simulink library "amg_sense_temphumid_lib"  (R2015b)
settings: Solver=ode45  StartTime=0.0  StopTime=10.0  RelTol=1e-3
libraries: simulink x24, waijung_soft_i2c_lib x2
settings Model: Creator=Krisada  LastModifiedBy=Aimagin
settings DataIOCC: SaveFormat=Array  SignalLoggingSaveFormat=ModelDataLogs
settings OptimizationCC: ExpressionDepthLimit=2147483647
settings DebuggingCC: UnderspecifiedInitializationDetection=Classic  MergeDetectMultiDrivingBlocksExec=none  SolverPrmCheckMsg=warning  FcnCallInpInsideContextMsg=UseLocalSettings  StateNameClashWarn=warning  StrictBusMsg=Warning
settings HardwareCC: ProdBitPerPointer=32  ProdLargestAtomicFloat=None  ProdIntDivRoundTo=Undefined  ProdEndianess=Unspecified  ProdWordSize=32  ProdHWDeviceType=32-bit Generic
settings GRTTargetCC: CombineOutputUpdateFcns=off  GRTInterface=on
settings ConfigComp: CovModelRefEnable=Off

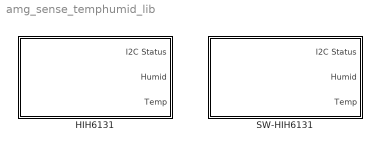
== system amg_sense_temphumid_lib ==
  HIH6131 : Subsystem  mask(stm32f4_i2c_sensors){module=1, slvaddr=hex2dec('4E'), outputlabel={'I2C Status','Humid (%)','Temp (C)'}, sensorname=STM32F4\naMG Sense - Temp/Humid, sampletime=0.5}
      mask prompts: module "I2C Module"; slvaddr "I2C Slave Address"; outputlabel "Output label"; sensorname "Sensor name"; sampletime "Sample time (sec)"
      mask help:
      | aMG Sense - Temp/Humid
      |
      | I2C Status:
      |  0 - Success
      |  1 - NAK
      |  2 - Timeout
      |  3 - Combined error, NAK+Timeout
      |
      | Note: Require I2C Setup block for the selected I2C module.
      mask init:
      | stm32f4_i2c_sensors_callback('init');
      mask TypeOptions module: 1 | 2 | 3
      mask Callback module: stm32f4_i2c_sensors_callback('module');
      mask Display: text(0.5, 0.5, 'STM32F4\naMG Sense - Temp/Humid','ver','middle','hor','center');port_label('output', 1,'I2C Status');port_label('output', 2,'Humid (%)');port_label('output', 3,'Temp (C)');
  SW-HIH6131 : Subsystem  mask(waijung_soft_i2c_sensors){module=1, slvaddr=hex2dec('4E'), outputlabel={'I2C Status','Humid (%)','Temp (C)'}, sensorname=Soft-I2C\naMG Sense - Temp/Humid, sampletime=0.5}
      mask prompts: module "I2C Module"; slvaddr "I2C Slave Address"; outputlabel "Output label"; sensorname "Sensor name"; sampletime "Sample time (sec)"
      mask help:
      | aMG Sense - Temp/Humid
      |
      | I2C Status:
      |  0 - Success
      |  1 - NAK
      |  2 - Timeout
      |  3 - Combined error, NAK+Timeout
      |
      | Note: Require I2C Setup block for the selected I2C module.
      mask init:
      | waijung_soft_i2c_sensors_callback('init');
      mask TypeOptions module: 1 | 2 | 3 | 4 | 5 | 6 | 7 | 8 | 9 | 10 | 11 | 12 | 13 | 14 | 15 | 16 | 17 | 18 | 19 | 20 | 21 | 22 | 23 | 24 | 25 | 26 | 27 | 28 | 29 | 30 | 31 | 32
      mask Callback module: waijung_soft_i2c_sensors_callback('module');
      mask Display: text(0.5, 0.5, 'Soft-I2C\naMG Sense - Temp/Humid','ver','middle','hor','center');port_label('output', 1,'I2C Status');port_label('output', 2,'Humid (%)');port_label('output', 3,'Temp (C)');

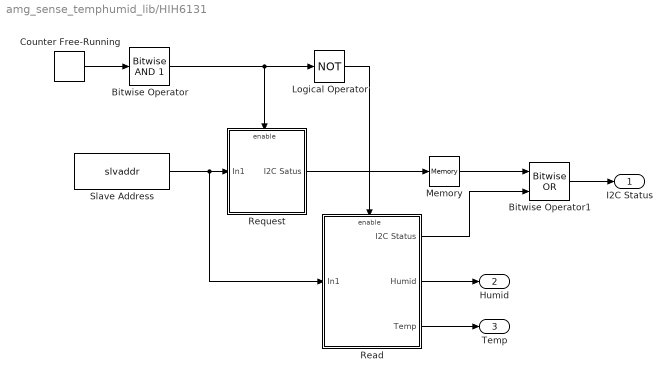
== system amg_sense_temphumid_lib/HIH6131 ==
  Bitwise Operator : simulink/Logic and Bit Operations/Bitwise Operator  logicop=AND  UseBitMask=on  BitMask=1  BitMaskRealWorld=Stored Integer
  Bitwise Operator1 : simulink/Logic and Bit Operations/Bitwise Operator  logicop=OR  UseBitMask=off  NumInputPorts=2  BitMask=bin2dec('11011001')  BitMaskRealWorld=Stored Integer
  Counter Free-Running : simulink/Sources/Counter Free-Running  SystemSampleTime=-1  NumBits=16  tsamp=-1
  Logical Operator : Logic  Operator=NOT  AllPortsSameDT=off  OutDataTypeStr=boolean
  Memory : Memory  InheritSampleTime=on  LinearizeMemory=on
  Read : Subsystem
  Request : Subsystem
  Slave Address : Constant  Value=slvaddr  OutDataTypeStr=uint8  SampleTime=sampletime
  I2C Status : Outport
  Humid : Outport  Port=2
  Temp : Outport  Port=3
  wires:
  Counter Free-Running/1 -> Bitwise Operator/1
  Bitwise Operator/1 -> Logical Operator/1, Request/Enable
  Logical Operator/1 -> Read/Enable
  Slave Address/1 -> Request/1(In1), Read/1(In1)
  Read/2(Humid) -> Humid/1
  Read/3(Temp) -> Temp/1
  Request/1(I2C Satus) -> Memory/1
  Memory/1 -> Bitwise Operator1/1
  Read/1(I2C Status) -> Bitwise Operator1/2
  Bitwise Operator1/1 -> I2C Status/1

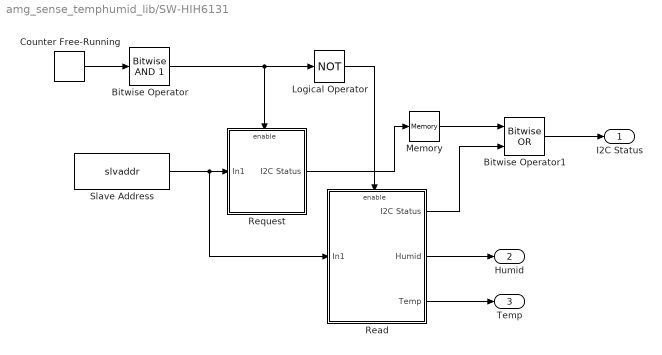
== system amg_sense_temphumid_lib/SW-HIH6131 ==
  Bitwise Operator : simulink/Logic and Bit Operations/Bitwise Operator  logicop=AND  UseBitMask=on  BitMask=1  BitMaskRealWorld=Stored Integer
  Bitwise Operator1 : simulink/Logic and Bit Operations/Bitwise Operator  logicop=OR  UseBitMask=off  NumInputPorts=2  BitMask=bin2dec('11011001')  BitMaskRealWorld=Stored Integer
  Counter Free-Running : simulink/Sources/Counter Free-Running  SystemSampleTime=-1  NumBits=16  tsamp=-1
  Logical Operator : Logic  Operator=NOT  AllPortsSameDT=off  OutDataTypeStr=boolean
  Memory : Memory  InheritSampleTime=on  LinearizeMemory=on
  Read : Subsystem
  Request : Subsystem
  Slave Address : Constant  Value=slvaddr  OutDataTypeStr=uint8  SampleTime=sampletime
  I2C Status : Outport
  Humid : Outport  Port=2
  Temp : Outport  Port=3
  wires:
  Read/3(Temp) -> Temp/1
  Read/2(Humid) -> Humid/1
  Slave Address/1 -> Read/1(In1), Request/1(In1)
  Logical Operator/1 -> Read/Enable
  Bitwise Operator/1 -> Request/Enable, Logical Operator/1
  Counter Free-Running/1 -> Bitwise Operator/1
  Request/1(I2C Status) -> Memory/1
  Memory/1 -> Bitwise Operator1/1
  Read/1(I2C Status) -> Bitwise Operator1/2
  Bitwise Operator1/1 -> I2C Status/1

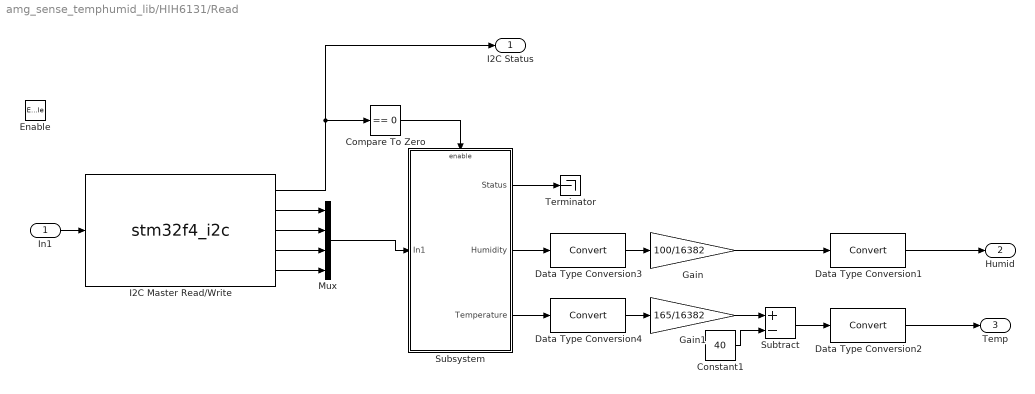
== system amg_sense_temphumid_lib/HIH6131/Read ==
  In1 : Inport
  Enable : EnablePort  PropagateVarSize=During execution
  Compare To Zero : simulink/Logic and Bit Operations/Compare To Zero  SystemSampleTime=-1  relop===  LogicOutDataTypeMode=boolean  ZeroCross=off
  Constant1 : Constant  Value=40
  Data Type Conversion{1..4} (4 alike) : DataTypeConversion
  Gain : Gain  Gain=100/16382
  Gain1 : Gain  Gain=165/16382
  I2C Master Read/Write : S-Function  FunctionName=stm32f4_i2c  Parameters=configuration,module,transfer,clkspeed,timeout,sdapin,sclpin,writecount,readcount,inputtypearray,outputtypearray,confstr,sampletime,sampletimestr,blockid  SFunctionDeploymentMode=off  EnableBusSupport=off  mask(stm32f4_i2c){configuration=Transaction, module=1, lastmodule=3, transfer=Blocking, dutycycle=TLow/THigh = 2, clkspeed=400, timeout=25, writecount=0, readcount=4, sdapin=C9, sclpin=A8, waitwritetime=0, inputtypearray=[1 3], outputtypearray=[5 3 3 3 3 3], confstr=["C","9","A","8","1","1","6","0","I2C_DutyCycle_2","0","off"], sampletime=-1, sampletimestr=0.5, blockid=ReadI2CMasterReadWrite}
      mask prompts: module "I2C Module"; lastmodule "Last module"; transfer "Transfer mode"; dutycycle "Duty cycle in fast mode"; clkspeed "Clock speed (kHz)"; timeout "Timeout (ms)"; writecount "Bytes write count"; readcount "Bytes read count"; sdapin "SDA pin"; sclpin "SCL pin"; waitwritetime "Wait write time (ms), default is 0"; inputtypearray "Input type array"; outputtypearray "Output type array"; confstr "Configuration string"; sampletime "Sample time (sec)"; sampletimestr "Compiled sample time (sec) in string"
      mask init:
      | stm32f4_i2c_callback('init');
      mask Help: web(fullfile(waijungdocroot,'stm32f4_i2c_readwrite.htm'), '-browser')
      mask TypeOptions configuration: Setup | Transaction
      mask Callback configuration: stm32f4_i2c_callback('configuration');
      mask TypeOptions module: 1 | 2 | 3
      mask Callback module: stm32f4_i2c_callback('module');
      mask TypeOptions transfer: Blocking | Non-blocking
      mask TypeOptions dutycycle: TLow/THigh = 16/9 | TLow/THigh = 2
      mask Callback dutycycle: stm32f4_i2c_callback('dutycycle');
      mask Callback writecount: stm32f4_i2c_callback('writecount');
      mask Callback readcount: stm32f4_i2c_callback('readcount');
      mask TypeOptions sdapin: - | C9
      mask Callback sdapin: stm32f4_i2c_callback('sdapin');
      mask TypeOptions sclpin: - | A8
      mask Callback sclpin: stm32f4_i2c_callback('sclpin');
      mask Callback confstr: stm32f4_i2c_callback('confstr');
      mask Callback sampletime: stm32f4_i2c_callback('sampletime');
      mask Callback sampletimestr: stm32f4_i2c_callback('sampletimestr');
      mask Callback blockid: stm32f4_i2c_callback('blockid');
      mask Display: text(0.5, 0.5, 'Module: I2C1\nTransfer: Blocking\nWrite: 0 bytes\nRead: 4 bytes\nTs (sec): 0.5','ver','middle','hor','center');port_label('input', 1,'SlvAddr');port_label('output', 1,'Status');port_label('output', 2,'Rd0 (uint8)');port_label('output', 3,'Rd1 (uint8)');port_label('output', 4,'Rd2 (uint8)');port_label('output', 5,'Rd3 (uint8)');
  Mux : Mux
  Subsystem : Subsystem
  Subtract : Sum  Inputs=+-
  Terminator : Terminator
  I2C Status : Outport
  Humid : Outport  Port=2
  Temp : Outport  Port=3
  wires:
  I2C Master Read/Write/2 -> Mux/1
  I2C Master Read/Write/3 -> Mux/2
  I2C Master Read/Write/4 -> Mux/3
  I2C Master Read/Write/5 -> Mux/4
  Mux/1 -> Subsystem/1(In1)
  Compare To Zero/1 -> Subsystem/Enable
  I2C Master Read/Write/1 -> Compare To Zero/1, I2C Status/1
  Subsystem/2(Humidity) -> Data Type Conversion3/1
  Subsystem/3(Temperature) -> Data Type Conversion4/1
  Gain1/1 -> Subtract/1
  Constant1/1 -> Subtract/2
  Subsystem/1(Status) -> Terminator/1
  Subtract/1 -> Data Type Conversion2/1
  Data Type Conversion3/1 -> Gain/1
  Data Type Conversion4/1 -> Gain1/1
  Gain/1 -> Data Type Conversion1/1
  Data Type Conversion1/1 -> Humid/1
  Data Type Conversion2/1 -> Temp/1
  In1/1 -> I2C Master Read/Write/1

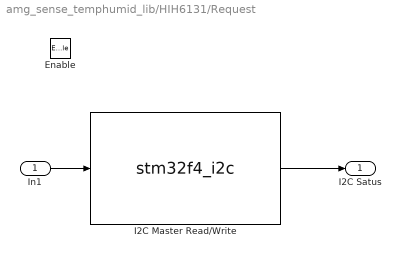
== system amg_sense_temphumid_lib/HIH6131/Request ==
  In1 : Inport
  Enable : EnablePort  PropagateVarSize=During execution
  I2C Master Read/Write : S-Function  FunctionName=stm32f4_i2c  Parameters=configuration,module,transfer,clkspeed,timeout,sdapin,sclpin,writecount,readcount,inputtypearray,outputtypearray,confstr,sampletime,sampletimestr,blockid  SFunctionDeploymentMode=off  EnableBusSupport=off  mask(stm32f4_i2c){configuration=Transaction, module=1, lastmodule=3, transfer=Blocking, dutycycle=TLow/THigh = 2, clkspeed=400, timeout=25, writecount=0, readcount=0, sdapin=C9, sclpin=A8, waitwritetime=0, inputtypearray=[1 3], outputtypearray=[1 3], confstr=["C","9","A","8","1","1","6","0","I2C_DutyCycle_2","0","off"], sampletime=-1, sampletimestr=0.5, blockid=RequestI2CMasterReadWrite}
      mask prompts: module "I2C Module"; lastmodule "Last module"; transfer "Transfer mode"; dutycycle "Duty cycle in fast mode"; clkspeed "Clock speed (kHz)"; timeout "Timeout (ms)"; writecount "Bytes write count"; readcount "Bytes read count"; sdapin "SDA pin"; sclpin "SCL pin"; waitwritetime "Wait write time (ms), default is 0"; inputtypearray "Input type array"; outputtypearray "Output type array"; confstr "Configuration string"; sampletime "Sample time (sec)"; sampletimestr "Compiled sample time (sec) in string"
      mask init:
      | stm32f4_i2c_callback('init');
      mask Help: web(fullfile(waijungdocroot,'stm32f4_i2c_readwrite.htm'), '-browser')
      mask TypeOptions configuration: Setup | Transaction
      mask Callback configuration: stm32f4_i2c_callback('configuration');
      mask TypeOptions module: 1 | 2 | 3
      mask Callback module: stm32f4_i2c_callback('module');
      mask TypeOptions transfer: Blocking | Non-blocking
      mask TypeOptions dutycycle: TLow/THigh = 16/9 | TLow/THigh = 2
      mask Callback dutycycle: stm32f4_i2c_callback('dutycycle');
      mask Callback writecount: stm32f4_i2c_callback('writecount');
      mask Callback readcount: stm32f4_i2c_callback('readcount');
      mask TypeOptions sdapin: - | C9
      mask Callback sdapin: stm32f4_i2c_callback('sdapin');
      mask TypeOptions sclpin: - | A8
      mask Callback sclpin: stm32f4_i2c_callback('sclpin');
      mask Callback confstr: stm32f4_i2c_callback('confstr');
      mask Callback sampletime: stm32f4_i2c_callback('sampletime');
      mask Callback sampletimestr: stm32f4_i2c_callback('sampletimestr');
      mask Callback blockid: stm32f4_i2c_callback('blockid');
      mask Display: text(0.5, 0.5, 'Module: I2C1\nTransfer: Blocking\nWrite: 0 bytes\nRead: 0 bytes\nTs (sec): 0.5','ver','middle','hor','center');port_label('input', 1,'SlvAddr');port_label('output', 1,'Status');
  I2C Satus : Outport
  wires:
  In1/1 -> I2C Master Read/Write/1
  I2C Master Read/Write/1 -> I2C Satus/1

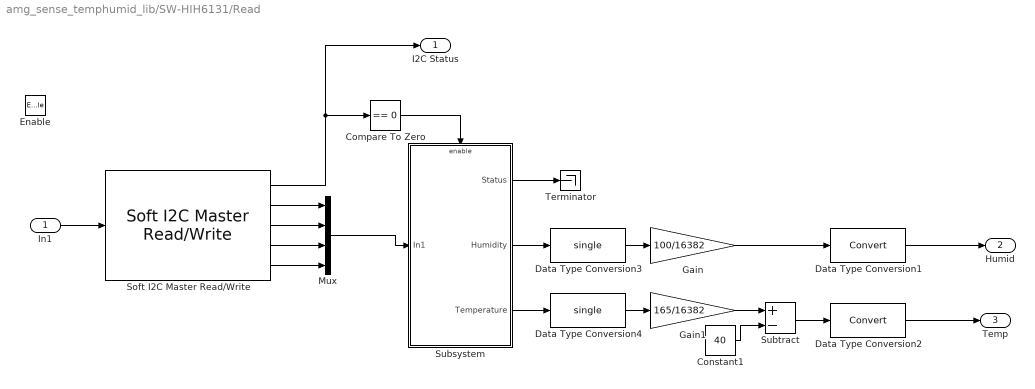
== system amg_sense_temphumid_lib/SW-HIH6131/Read ==
  In1 : Inport
  Enable : EnablePort  PropagateVarSize=During execution
  Compare To Zero : simulink/Logic and Bit Operations/Compare To Zero  SystemSampleTime=-1  relop===  LogicOutDataTypeMode=boolean  ZeroCross=off
  Constant1 : Constant  Value=40  OutDataTypeStr=single
  Data Type Conversion1 : DataTypeConversion
  Data Type Conversion2 : DataTypeConversion
  Data Type Conversion3 : DataTypeConversion  OutDataTypeStr=single
  Data Type Conversion4 : DataTypeConversion  OutDataTypeStr=single
  Gain : Gain  Gain=100/16382
  Gain1 : Gain  Gain=165/16382
  Mux : Mux
  Soft I2C Master Read/Write : waijung_soft_i2c_lib/Soft I2C Master Read//Write  conf=ReadWrite  targetname=0  module=1  transfer=Blocking  clk=100  timeout=25  sdapins={'A4','A6'}  sclpins='A5'  writecount=0  readcount=4  waittime=0  forcestop=off  portpinstr=0  sampletime=inf  blockid=SWHIH6131ReadSoftI2CMasterReadWrite  inputporttype=[3]  inputportwidth=[]  inputportlabel={'SlvAddr'}  outputporttype=[3 3 3 3 3]  outputportwidth=[1 1 1 1 1]  outputportlabel={'Status' 'Rd0 (uint8)' 'Rd1 (uint8)' 'Rd2 (uint8)' 'Rd3 (uint8)'}  compat=0  optionstring=[]
  Subsystem : Subsystem
  Subtract : Sum  Inputs=+-
  Terminator : Terminator
  I2C Status : Outport
  Humid : Outport  Port=2
  Temp : Outport  Port=3
  wires:
  In1/1 -> Soft I2C Master Read/Write/1
  Data Type Conversion2/1 -> Temp/1
  Data Type Conversion1/1 -> Humid/1
  Gain/1 -> Data Type Conversion1/1
  Data Type Conversion4/1 -> Gain1/1
  Data Type Conversion3/1 -> Gain/1
  Subtract/1 -> Data Type Conversion2/1
  Subsystem/1(Status) -> Terminator/1
  Constant1/1 -> Subtract/2
  Gain1/1 -> Subtract/1
  Subsystem/3(Temperature) -> Data Type Conversion4/1
  Subsystem/2(Humidity) -> Data Type Conversion3/1
  Soft I2C Master Read/Write/1 -> Compare To Zero/1, I2C Status/1
  Compare To Zero/1 -> Subsystem/Enable
  Mux/1 -> Subsystem/1(In1)
  Soft I2C Master Read/Write/5 -> Mux/4
  Soft I2C Master Read/Write/4 -> Mux/3
  Soft I2C Master Read/Write/3 -> Mux/2
  Soft I2C Master Read/Write/2 -> Mux/1

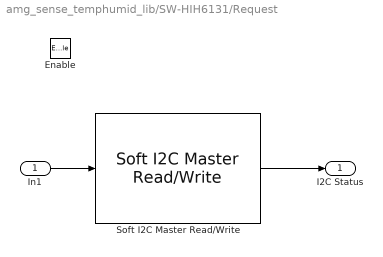
== system amg_sense_temphumid_lib/SW-HIH6131/Request ==
  In1 : Inport
  Enable : EnablePort  PropagateVarSize=During execution
  Soft I2C Master Read/Write : waijung_soft_i2c_lib/Soft I2C Master Read//Write  conf=ReadWrite  targetname=0  module=1  transfer=Blocking  clk=100  timeout=25  sdapins={'A4','A6'}  sclpins='A5'  writecount=0  readcount=0  waittime=0  forcestop=off  portpinstr=0  sampletime=inf  blockid=SWHIH6131RequestSoftI2CMasterReadWrite  inputporttype=[3]  inputportwidth=[]  inputportlabel={'SlvAddr'}  outputporttype=[3]  outputportwidth=[1]  outputportlabel={'Status'}  compat=0  optionstring=[]
  I2C Status : Outport
  wires:
  Soft I2C Master Read/Write/1 -> I2C Status/1
  In1/1 -> Soft I2C Master Read/Write/1

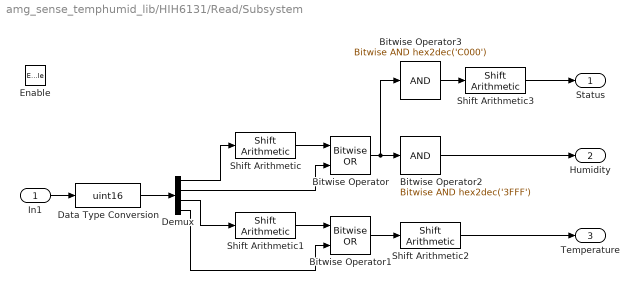
== system amg_sense_temphumid_lib/HIH6131/Read/Subsystem ==
  In1 : Inport
  Enable : EnablePort  PropagateVarSize=During execution
  Bitwise Operator : simulink/Logic and Bit Operations/Bitwise Operator  logicop=OR  UseBitMask=off  NumInputPorts=2  BitMask=bin2dec('11011001')  BitMaskRealWorld=Stored Integer
  Bitwise Operator1 : simulink/Logic and Bit Operations/Bitwise Operator  logicop=OR  UseBitMask=off  NumInputPorts=2  BitMask=bin2dec('11011001')  BitMaskRealWorld=Stored Integer
  Bitwise Operator2 : simulink/Logic and Bit Operations/Bitwise Operator  logicop=AND  UseBitMask=on  BitMask=hex2dec('3FFF')  BitMaskRealWorld=Stored Integer
  Bitwise Operator3 : simulink/Logic and Bit Operations/Bitwise Operator  logicop=AND  UseBitMask=on  BitMask=hex2dec('C000')  BitMaskRealWorld=Stored Integer
  Data Type Conversion : DataTypeConversion  OutDataTypeStr=uint16
  Demux : Demux
  Shift Arithmetic : simulink/Logic and Bit Operations/Shift Arithmetic  SystemSampleTime=-1  nBitShiftRight=-8  nBinPtShiftRight=0
  Shift Arithmetic1 : simulink/Logic and Bit Operations/Shift Arithmetic  SystemSampleTime=-1  nBitShiftRight=-8  nBinPtShiftRight=0
  Shift Arithmetic2 : simulink/Logic and Bit Operations/Shift Arithmetic  SystemSampleTime=-1  nBitShiftRight=2  nBinPtShiftRight=0
  Shift Arithmetic3 : simulink/Logic and Bit Operations/Shift Arithmetic  SystemSampleTime=-1  nBitShiftRight=14  nBinPtShiftRight=0
  Status : Outport
  Humidity : Outport  Port=2
  Temperature : Outport  Port=3
  wires:
  Data Type Conversion/1 -> Demux/1
  Demux/1 -> Shift Arithmetic/1
  Shift Arithmetic/1 -> Bitwise Operator/1
  Demux/2 -> Bitwise Operator/2
  Demux/3 -> Shift Arithmetic1/1
  Shift Arithmetic1/1 -> Bitwise Operator1/1
  Demux/4 -> Bitwise Operator1/2
  Bitwise Operator/1 -> Bitwise Operator2/1, Bitwise Operator3/1
  Bitwise Operator1/1 -> Shift Arithmetic2/1
  Bitwise Operator3/1 -> Shift Arithmetic3/1
  Shift Arithmetic3/1 -> Status/1
  Bitwise Operator2/1 -> Humidity/1
  In1/1 -> Data Type Conversion/1
  Shift Arithmetic2/1 -> Temperature/1

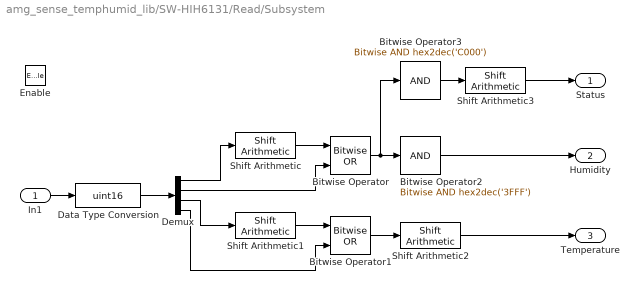
== system amg_sense_temphumid_lib/SW-HIH6131/Read/Subsystem ==
  In1 : Inport
  Enable : EnablePort  PropagateVarSize=During execution
  Bitwise Operator : simulink/Logic and Bit Operations/Bitwise Operator  logicop=OR  UseBitMask=off  NumInputPorts=2  BitMask=bin2dec('11011001')  BitMaskRealWorld=Stored Integer
  Bitwise Operator1 : simulink/Logic and Bit Operations/Bitwise Operator  logicop=OR  UseBitMask=off  NumInputPorts=2  BitMask=bin2dec('11011001')  BitMaskRealWorld=Stored Integer
  Bitwise Operator2 : simulink/Logic and Bit Operations/Bitwise Operator  logicop=AND  UseBitMask=on  BitMask=hex2dec('3FFF')  BitMaskRealWorld=Stored Integer
  Bitwise Operator3 : simulink/Logic and Bit Operations/Bitwise Operator  logicop=AND  UseBitMask=on  BitMask=hex2dec('C000')  BitMaskRealWorld=Stored Integer
  Data Type Conversion : DataTypeConversion  OutDataTypeStr=uint16
  Demux : Demux
  Shift Arithmetic : simulink/Logic and Bit Operations/Shift Arithmetic  SystemSampleTime=-1  nBitShiftRight=-8  nBinPtShiftRight=0
  Shift Arithmetic1 : simulink/Logic and Bit Operations/Shift Arithmetic  SystemSampleTime=-1  nBitShiftRight=-8  nBinPtShiftRight=0
  Shift Arithmetic2 : simulink/Logic and Bit Operations/Shift Arithmetic  SystemSampleTime=-1  nBitShiftRight=2  nBinPtShiftRight=0
  Shift Arithmetic3 : simulink/Logic and Bit Operations/Shift Arithmetic  SystemSampleTime=-1  nBitShiftRight=14  nBinPtShiftRight=0
  Status : Outport
  Humidity : Outport  Port=2
  Temperature : Outport  Port=3
  wires:
  Shift Arithmetic2/1 -> Temperature/1
  In1/1 -> Data Type Conversion/1
  Bitwise Operator2/1 -> Humidity/1
  Shift Arithmetic3/1 -> Status/1
  Bitwise Operator3/1 -> Shift Arithmetic3/1
  Bitwise Operator1/1 -> Shift Arithmetic2/1
  Bitwise Operator/1 -> Bitwise Operator3/1, Bitwise Operator2/1
  Demux/4 -> Bitwise Operator1/2
  Shift Arithmetic1/1 -> Bitwise Operator1/1
  Demux/3 -> Shift Arithmetic1/1
  Demux/2 -> Bitwise Operator/2
  Shift Arithmetic/1 -> Bitwise Operator/1
  Demux/1 -> Shift Arithmetic/1
  Data Type Conversion/1 -> Demux/1
